simulink model "BO_Q2"  (R2025b)
settings: Solver=VariableStepAuto  StartTime=0.0  StopTime=400  RelTol=1e-3
undefined symbols (not defined in the file): Gb, Ib, n, p1, p2, p3, x0
settings Model: Creator=Louis  LastModifiedBy=Louis

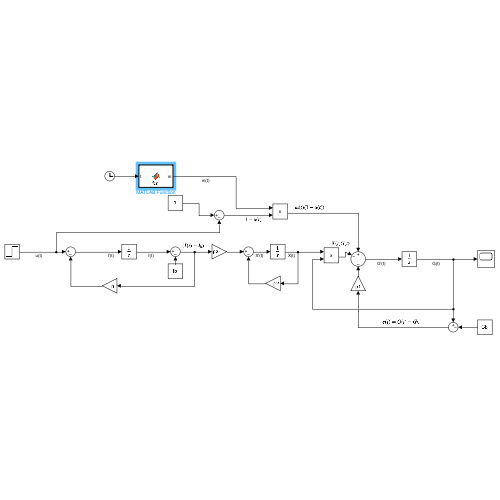
[thumbnail: Simulink's stored preview of the top-level diagram]
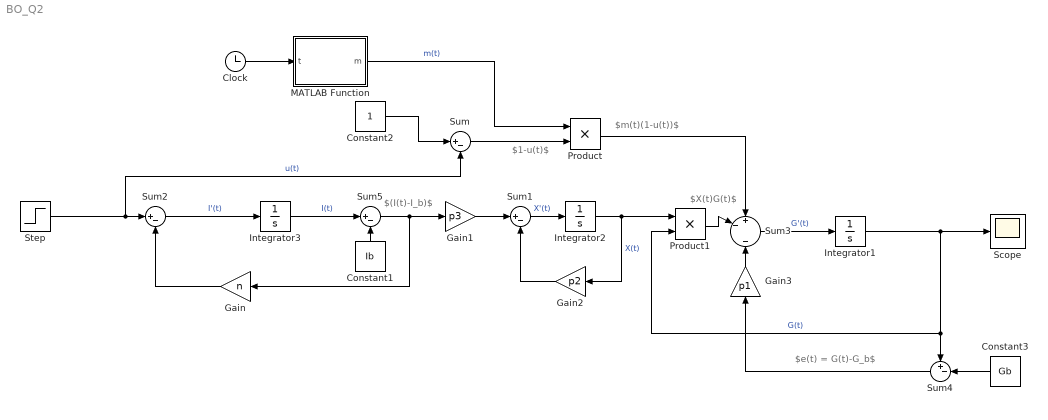
== system BO_Q2 ==
  note: $X(t)G(t)$
  note: $1-u(t)$
  note: $m(t)(1-u(t))$
  note: $(I(t)-I_b)$
  note: $e(t) = G(t)-G_b$
  Clock : Clock
  Constant1 : Constant  Value=Ib
  Constant2 : Constant
  Constant3 : Constant  Value=Gb
  Gain : Gain  Gain=n
  Gain1 : Gain  Gain=p3
  Gain2 : Gain  Gain=p2
  Gain3 : Gain  Gain=p1
  Integrator1 : Integrator  InitialCondition=x0(1)
  Integrator2 : Integrator  InitialCondition=x0(2)
  Integrator3 : Integrator  InitialCondition=x0(3)
  MATLAB Function : MATLAB Function  TreatAsAtomicUnit=on
  Product : Product
  Product1 : Product
  Scope : Scope
      settings: ActiveDisplayYMinimum=-1  ActiveDisplayYMaximum=1  DataLoggingVariableName=GBO_Q2  DataLoggingSaveFormat=Array
  Step : Step  Time=0  After=2  SampleTime=0
  Sum{,1..2,5} (4 alike) : Sum  Inputs=|+-
  Sum3 : Sum  Inputs=+-|-
  Sum4 : Sum  Inputs=+-|
  wires:
  Product/1 -> Sum3/1
  Sum4/1 -> Gain3/1
  Gain/1 -> Sum2/2
  Integrator2/1 -> Product1/1, Gain2/1  "X(t)"
  Constant2/1 -> Sum/1
  Integrator1/1 -> Scope/1, Sum4/1, Product1/2  "G(t)"
  Integrator3/1 -> Sum5/1  "I(t)"
  Product1/1 -> Sum3/2
  Constant1/1 -> Sum5/2
  Gain1/1 -> Sum1/1
  Gain2/1 -> Sum1/2
  MATLAB Function/1(m) -> Product/1  "m(t)"
  Sum1/1 -> Integrator2/1  "X'(t)"
  Gain3/1 -> Sum3/3
  Sum5/1 -> Gain/1, Gain1/1
  Constant3/1 -> Sum4/2
  Sum3/1 -> Integrator1/1  "G'(t)"
  Sum2/1 -> Integrator3/1  "I'(t)"
  Sum/1 -> Product/2
  Step/1 -> Sum2/1, Sum/2  "u(t)"
  Clock/1 -> MATLAB Function/1(t)

== matlab function BO_Q2/MATLAB Function ==
  data: t input; m output
function m = fcn(t)

if (t <= 0 && t >= 5)
    m = 5*1;

else
    m = 0;
end
